simulink subsystem "controller"  (R2023b)
settings: Solver=VariableStepAuto  StartTime=0.0  StopTime=10.0  RelTol=1e-3
undefined symbols (not defined in the file or in its folder): tau_s
settings Model: Creator=Previ  LastModifiedBy=Previ

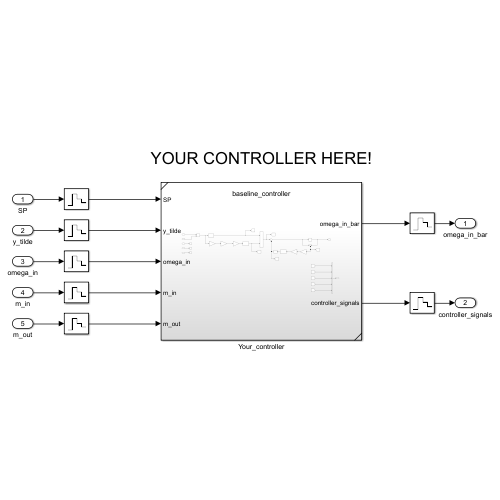
[thumbnail: Simulink's stored preview of the top-level diagram]
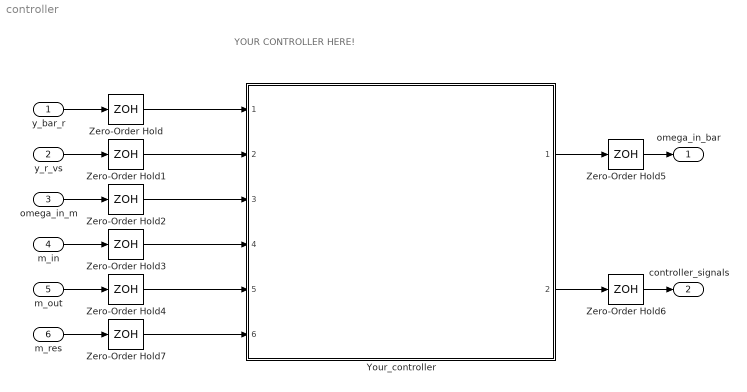
== system controller ==
  note: YOUR CONTROLLER HERE!
  y_bar_r : Inport  PortDimensions=[1, 1]
  y_r_vs : Inport  Port=2  PortDimensions=[1, 1]
  omega_in_m : Inport  Port=3  PortDimensions=[1, 1]
  m_in : Inport  Port=4  PortDimensions=[1, 1]
  m_out : Inport  Port=5  PortDimensions=[1, 1]
  m_res : Inport  Port=6  PortDimensions=[1, 1]
  Your_controller : Subsystem  ReferencedSubsystem=baseline_controller
  Zero-Order Hold{,1..7} (8 alike) : ZeroOrderHold  SampleTime=tau_s
  omega_in_bar : Outport  PortDimensions=[1, 1]
  controller_signals : Outport  Port=2
  wires:
  y_bar_r/1 -> Zero-Order Hold/1
  y_r_vs/1 -> Zero-Order Hold1/1
  omega_in_m/1 -> Zero-Order Hold2/1
  m_in/1 -> Zero-Order Hold3/1
  m_out/1 -> Zero-Order Hold4/1
  Zero-Order Hold5/1 -> omega_in_bar/1
  Zero-Order Hold6/1 -> controller_signals/1
  Zero-Order Hold/1 -> Your_controller/1
  Zero-Order Hold1/1 -> Your_controller/2
  Zero-Order Hold2/1 -> Your_controller/3
  Zero-Order Hold4/1 -> Your_controller/5
  Zero-Order Hold3/1 -> Your_controller/4
  Your_controller/2 -> Zero-Order Hold6/1
  Your_controller/1 -> Zero-Order Hold5/1
  m_res/1 -> Zero-Order Hold7/1
  Zero-Order Hold7/1 -> Your_controller/6
